simulink model "Vagolap"  (Simulink 8.3)
settings: Solver=ode45  StartTime=0.0  StopTime=10.0  RelTol=1e-3
values from neighbouring files (symbols this model uses):
  Butterworth_filter_order = 8    [Sketch_controller_model_ini.m]    (also in Symmetry_REAL_TIME_ini.m; Symmetry_ini.m)
  sample = 10e-5    (= 0.0001)    [Inverter_ini.m]    (also in Sketch_controller_model_ini.m; Symmetry_REAL_TIME_ini.m; Symmetry_ini.m; Symmetry_ini_COPY.m)
libraries: powerlib x4, dsparch4 x3
settings Model: Creator=Templomos  LastModifiedBy=Templomos
settings DataIOCC: SignalLoggingSaveFormat=Dataset
settings DebuggingCC: UnderspecifiedInitializationDetection=Simplified  StateNameClashWarn=none
settings GRTTargetCC: CombineOutputUpdateFcns=on  GRTInterface=off

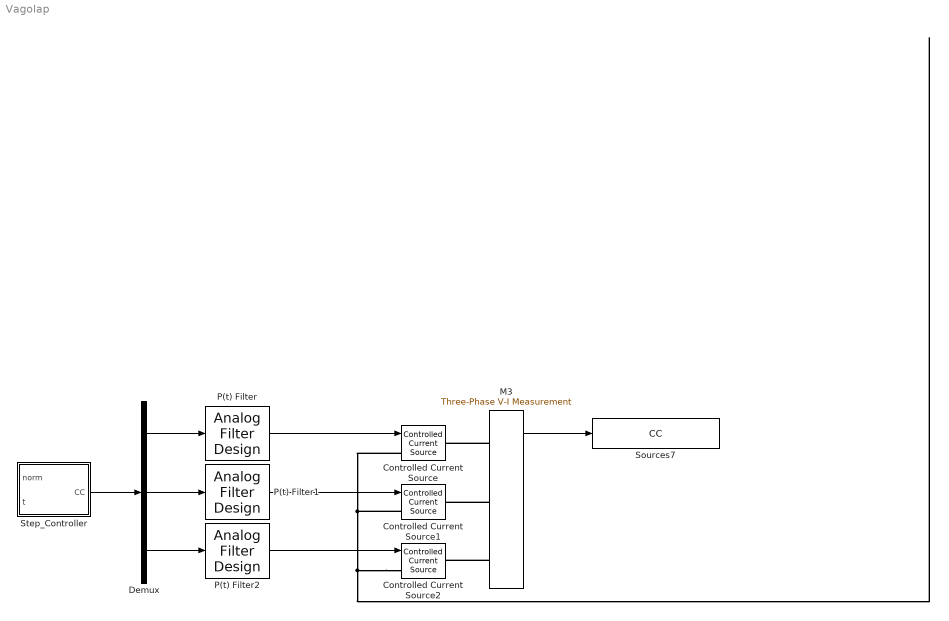
== system Vagolap ==
  Controlled Current Source : powerlib/Electrical Sources/Controlled Current Source  Initialize=on  Source_Type=AC  Amplitude=0  Phase=0  Frequency=0  Measurements=None
  Controlled Current Source1 : powerlib/Electrical Sources/Controlled Current Source  Initialize=on  Source_Type=AC  Amplitude=0  Phase=0  Frequency=0  Measurements=None
  Controlled Current Source2 : powerlib/Electrical Sources/Controlled Current Source  Initialize=on  Source_Type=AC  Amplitude=0  Phase=0  Frequency=0  Measurements=None
  Demux : Demux  Outputs=3
  M3 : powerlib/Measurements/Three-Phase V-I Measurement  VoltageMeasurement=no  SetLabelV=off  LabelV=V_RST  Vpu=off  VpuLL=off  CurrentMeasurement=yes  SetLabelI=off  LabelI=I_RST  Ipu=off  Pbase=100e6  Vbase=500e3  OutputType=Complex  PhasorSimulation=off  PSBequivalent=0
  P(t) Filter : dsparch4/Analog Filter Design  method=Butterworth  filttype=Lowpass  N=Butterworth_filter_order  Wlo=Butterworth_passband_frequency  Whi=80  Rp=2  Rs=40
  P(t) Filter1 : dsparch4/Analog Filter Design  method=Butterworth  filttype=Lowpass  N=Butterworth_filter_order  Wlo=Butterworth_passband_frequency  Whi=80  Rp=2  Rs=40
  P(t) Filter2 : dsparch4/Analog Filter Design  method=Butterworth  filttype=Lowpass  N=Butterworth_filter_order  Wlo=Butterworth_passband_frequency  Whi=80  Rp=2  Rs=40
  Sources7 : ToWorkspace  VariableName=CC  SaveFormat=Structure With Time  SampleTime=sample
  Step_Controller : MATLAB Function  TreatAsAtomicUnit=on
  wires:
  ? -> Step_Controller/1(norm)
  Step_Controller/1(CC) -> Demux/1
  M3/1 -> Sources7/1
  P(t) Filter2/1 -> Controlled Current Source2/1
  Demux/1 -> P(t) Filter/1
  Demux/2 -> P(t) Filter1/1
  P(t) Filter1/1 -> Controlled Current Source1/1
  P(t) Filter/1 -> Controlled Current Source/1
  Demux/3 -> P(t) Filter2/1
  ? -> Step_Controller/2(t)
  connections:
  Controlled Current Source2/LConn1 -- Controlled Current Source/LConn1 -- Controlled Current Source1/LConn1
  M3/LConn2 -- Controlled Current Source1/RConn1
  M3/LConn3 -- Controlled Current Source2/RConn1
  M3/LConn1 -- Controlled Current Source/RConn1

== matlab function Step_Controller ==
  data: norm input double; CC output double; t input double
function CC= fcn(norm,t)
%#codegen



Control_Current_frequency=[20,     30,     40];       %[Hz]
Control_Current_Amplitude=[0,     0,     0];       %[A]
Control_Current_Phase=    [0,      2/3*pi, 4/3*pi];   %[rad]
Control_Current_DC=       [0,      0,      0];        %[A]

CC_mtx=[Control_Current_Amplitude', Control_Current_frequency',...
            Control_Current_Phase', Control_Current_DC'];
        
CC=[CC_mtx(1,1)*sin(2*pi*CC_mtx(1,2)*t+CC_mtx(1,3))+CC_mtx(1,4),...
    CC_mtx(2,1)*sin(2*pi*CC_mtx(2,2)*t+CC_mtx(2,3))+CC_mtx(2,4),...
    CC_mtx(3,1)*sin(2*pi*CC_mtx(3,2)*t+CC_mtx(3,3))+CC_mtx(3,4)];
